simulink model "hw2_1"  (R2018a)
settings: Solver=VariableStepAuto  StartTime=0.0  StopTime=10.0  RelTol=1e-3
libraries: slctrlblks x1, dspsrcs4 x1
settings Model: Creator=kamil  LastModifiedBy=kamil

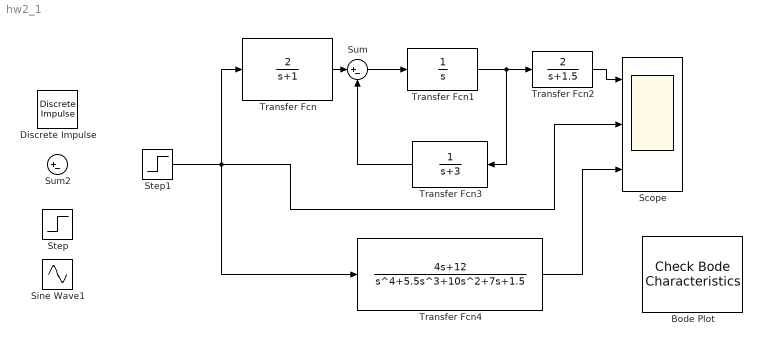
== system hw2_1 ==
  Bode Plot : slctrlblks/Model Verification/Check Bode  Characteristics  InstantiateOnLoad=on  SaveOperatingPoints=off  LinearizationIOs={'/Step1', 1, 'in', 'off', '';'/Transfer Fcn4', 1, 'out', 'on', ''}  LinearizeAt=SnapshotTimes  SnapshotTimes=[0]  TriggerType=rising  SampleTime=auto  RateConversionMethod=zoh  PreWarpFreq=10  UseExactDelayModel=off  UseFullBlockNameLabels=off  UseBusSignalLabels=off  enabled=on  stopWhenAssertionFail=off  export=off  ViewDlgPos=[1142 305 510 390]  OpenViewOnLoad=on  LaunchViewOnOpen=off  FrequencyUnits=rad/s  MagnitudeUnits=dB  PhaseUnits=deg  TimeUnits=seconds  EnableUpperBound=off  UpperBoundFrequencies=[]  UpperBoundMagnitudes=[]  EnableLowerBound=off  LowerBoundFrequencies=[]  LowerBoundMagnitudes=[]
      settings: SourceProductName=Simulink Control Design  SaveToWorkspace=on
  Discrete Impulse : dspsrcs4/Discrete  Impulse  Delay=0  SampleTime=1  FrameSample=1  OutputFrames=off  dataType=double  isSigned=on  wordLen=16  udDataType=sfix(16)  fracBitsMode=Best precision  numFracBits=15  OutDataTypeStr=double  LastOutDataTypeStr=double
  Scope : Scope  NumInputPorts=3
  Sine Wave1 : Sin  SampleTime=0
  Step : Step  Time=3  SampleTime=0
  Step1 : Step  SampleTime=0
  Sum : Sum  Inputs=|+-
  Sum2 : Sum  Inputs=|+-
  Transfer Fcn : TransferFcn  Numerator=[2]  Denominator=[1 1]
  Transfer Fcn1 : TransferFcn  Denominator=[1 0]
  Transfer Fcn2 : TransferFcn  Numerator=[2]  Denominator=[1 1.5]
  Transfer Fcn3 : TransferFcn  Denominator=[1 3]
  Transfer Fcn4 : TransferFcn  Numerator=[4 12]  Denominator=[1 5.5 10 7 1.5]
  wires:
  Transfer Fcn/1 -> Sum/1
  Sum/1 -> Transfer Fcn1/1
  Transfer Fcn1/1 -> Transfer Fcn3/1, Transfer Fcn2/1
  Transfer Fcn3/1 -> Sum/2
  Transfer Fcn4/1 -> Scope/3
  Transfer Fcn2/1 -> Scope/1
  Step1/1 -> Transfer Fcn4/1, Scope/2, Transfer Fcn/1
